simulink model "mrsRobotDetectorModel"  (R2019a)
settings: Solver=VariableStepAuto  StartTime=0.0  StopTime=10.0  RelTol=1e-3
libraries: mobileRoboticsLib x7
settings Model: Creator=scastro  LastModifiedBy=scastro
settings DataIOCC: ReturnWorkspaceOutputs=off
settings DebuggingCC: PregeneratedLibrarySubsystemCodeDiagnostic=none  ArithmeticOperatorsInVariantConditions=warning
settings SFSimCC: SimUseLocalCustomCode=off
settings RTWCC: RTWUseLocalCustomCode=off

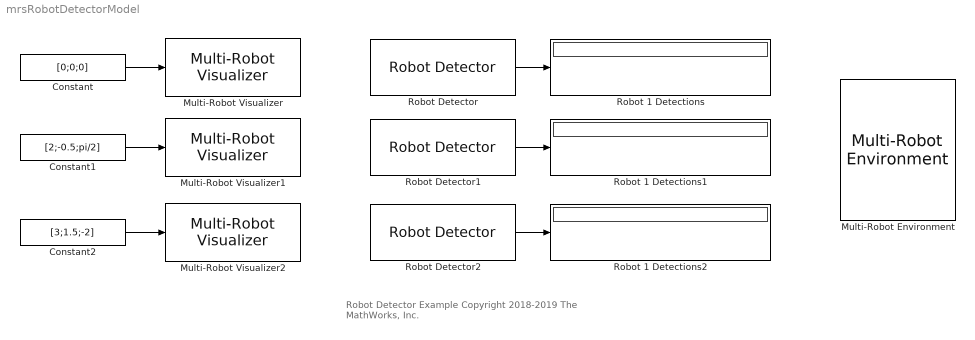
== system mrsRobotDetectorModel ==
  note: Robot Detector Example
      |
      | Copyright 2018-2019 The MathWorks, Inc.
  Constant : Constant  Value=[0;0;0]
  Constant1 : Constant  Value=[2;-0.5;pi/2]
  Constant2 : Constant  Value=[3;1.5;-2]
  Multi-Robot Environment : mobileRoboticsLib/Environments/Multi-Robot Environment  numRobots=3  showWaypoints=off  showObjects=off  objectColors=[ 1, 0, 0; 0, 1, 0; 0, 0, 1 ]  objectMarkers='s'  showRobotIds=on  plotSensorLines=on
      settings: SourceProductName=Mobile Robotics Simulation Toolbox
  Multi-Robot Visualizer : mobileRoboticsLib/Environments/Multi-Robot Visualizer  idx=1  radius=0  robotColor=[0 0 1]  showTraj=off  hasLidar=off  sensorOffset=[ 0, 0 ]  scanAngles=[ -pi/4, 0, pi/4 ]  maxNumScans=0  hasObjDetector=off  objDetectorOffset=[ 0, 0 ]  objDetectorAngle=0  objDetectorFOV=pi/3  objDetectorMaxRange=5  hasRobotDetector=on  robotDetectorOffset=[0,0]  robotDetectorAngle=0  robotDetectorFOV=pi/3  robotDetectorMaxRange=5  robotDetectorNumDetections=0
      settings: SourceProductName=Mobile Robotics Simulation Toolbox
  Multi-Robot Visualizer1 : mobileRoboticsLib/Environments/Multi-Robot Visualizer  idx=2  radius=0  robotColor=[0 0 1]  showTraj=off  hasLidar=off  sensorOffset=[ 0, 0 ]  scanAngles=[ -pi/4, 0, pi/4 ]  maxNumScans=0  hasObjDetector=off  objDetectorOffset=[ 0, 0 ]  objDetectorAngle=0  objDetectorFOV=pi/3  objDetectorMaxRange=5  hasRobotDetector=on  robotDetectorOffset=[0,0]  robotDetectorAngle=0  robotDetectorFOV=pi/3  robotDetectorMaxRange=5  robotDetectorNumDetections=0
      settings: SourceProductName=Mobile Robotics Simulation Toolbox
  Multi-Robot Visualizer2 : mobileRoboticsLib/Environments/Multi-Robot Visualizer  idx=3  radius=0  robotColor=[0 0 1]  showTraj=off  hasLidar=off  sensorOffset=[ 0, 0 ]  scanAngles=[ -pi/4, 0, pi/4 ]  maxNumScans=0  hasObjDetector=off  objDetectorOffset=[ 0, 0 ]  objDetectorAngle=0  objDetectorFOV=pi/3  objDetectorMaxRange=5  hasRobotDetector=on  robotDetectorOffset=[0,0]  robotDetectorAngle=0  robotDetectorFOV=pi/3  robotDetectorMaxRange=5  robotDetectorNumDetections=0
      settings: SourceProductName=Mobile Robotics Simulation Toolbox
  Robot 1 Detections : Display
  Robot 1 Detections1 : Display
  Robot 1 Detections2 : Display
  Robot Detector : mobileRoboticsLib/Environments/Robot Detector  robotIdx=1  sensorOffset=[ 0, 0 ]  sensorAngle=0  sensorFOV=pi/3  maxRange=5  maxDetections=3  sampleTime=0.1
      settings: SourceProductName=Mobile Robotics Simulation Toolbox
  Robot Detector1 : mobileRoboticsLib/Environments/Robot Detector  robotIdx=2  sensorOffset=[ 0, 0 ]  sensorAngle=0  sensorFOV=pi/3  maxRange=5  maxDetections=3  sampleTime=0.1
      settings: SourceProductName=Mobile Robotics Simulation Toolbox
  Robot Detector2 : mobileRoboticsLib/Environments/Robot Detector  robotIdx=3  sensorOffset=[ 0, 0 ]  sensorAngle=0  sensorFOV=pi/3  maxRange=5  maxDetections=3  sampleTime=0.1
      settings: SourceProductName=Mobile Robotics Simulation Toolbox
  wires:
  Robot Detector/1 -> Robot 1 Detections/1
  Constant/1 -> Multi-Robot Visualizer/1
  Constant1/1 -> Multi-Robot Visualizer1/1
  Constant2/1 -> Multi-Robot Visualizer2/1
  Robot Detector1/1 -> Robot 1 Detections1/1
  Robot Detector2/1 -> Robot 1 Detections2/1
